simulink model "RotateVideo"  (Simulink 6.4)
settings: Solver=ode45  StartTime=0.0  StopTime=5  RelTol=1e-3
undefined symbols (not defined in the file): jet
libraries: dspswit3 x1, dspwin32 x1, vipgeotforms x1, vipsnks x1
settings Model: LastModifiedBy=Pr . Saddam&Ali

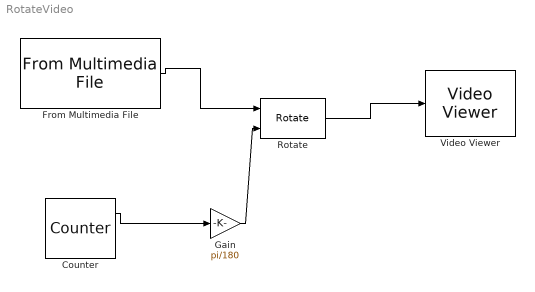
== system RotateVideo ==
  Counter : dspswit3/Counter  Direction=Up  CountEvent=Free running  CounterSize=User defined  MaxCount=255  InitialCount=1  Output=Count and Hit  HitValue=32  ResetInput=on  SamplesPerFrame=1  Ts=30  CntDtype=single  HitDtype=Logical
  From Multimedia File : dspwin32/From Multimedia File  DialogController=dspDDGCreate  DialogControllerArgs=DataTag0  inputFilename=vipmen.avi  loop=on  numPlays=inf  outputStreams=Video and audio  videoDataType=single  audioDataType=int16  inheritSampleTime=on  userDefinedSampleTime=1/30  noAudioOutput=off  isIntensityVideo=on  outputEOF=off
  Gain : Gain  Gain=pi/180  SampleTime=30
  Rotate : vipgeotforms/Rotate  DialogController=vipDDGCreate  DialogControllerArgs=DataTag1  outSizeR=Expanded to fit rotated input image  src_angle=Input port  unit_angle=Degrees  angle=100*pi/6  maxAngle=pi  dispImage=Center  method=Table lookup  interpMethod=Bilinear  prodOutputMode=Binary point scaling  prodOutputWordLength=32  prodOutputFracLength=10  roundingMode=Nearest  overflowMode=on
  Video Viewer : vipsnks/Video Viewer  inputType=Intensity  useColorMap=off  colormapValue=jet(256);  specRange=off  minInputVal=0  maxInputVal=255  FigPos=[411 355 203 203]  AxisZoom=on  trueSizedOnce=on
  wires:
  Counter/1 -> Gain/1
  Gain/1 -> Rotate/2
  From Multimedia File/1 -> Rotate/1
  Rotate/1 -> Video Viewer/1
